simulink model "TrafficLight"  (R2021a)
settings: Solver=FixedStepDiscrete  StartTime=0.0  StopTime=inf  RelTol=1e-3
settings Model: Creator=U3  LastModifiedBy=U3
settings OptimizationCC: DefaultParameterBehavior=Inlined  EnhancedBackFolding=on  PassReuseOutputArgsAs=Individual arguments  ZeroExternalMemoryAtStartup=off  ZeroInternalMemoryAtStartup=off  OptimizeBlockOrder=speed  DifferentSizesBufferReuse=on  OptimizationCustomize=off  EfficientTunableParamExpr=on
settings DebuggingCC: UnderspecifiedInitializationDetection=Classic  MergeDetectMultiDrivingBlocksExec=none  ParameterTunabilityLossMsg=error
settings ModelReferenceCC: PropagateSignalLabelsOutOfModel=off
settings SFSimCC: MATLABDynamicMemAlloc=off
settings RTWCC: SystemTargetFile=ert.tlc  GenCodeOnly=on  TemplateMakefile=ert_default_tmf  GenerateReport=on  IncludeHyperlinkInReport=on  LaunchReport=on  GenerateTraceInfo=on  GenerateTraceReport=on  GenerateTraceReportSl=on  GenerateTraceReportSf=on  GenerateTraceReportEml=on
settings CodeAppCC: ForceParamTrailComments=on  IgnoreCustomStorageClasses=off  OperatorAnnotations=on  SimulinkDataObjDesc=on  SFDataObjDesc=on  InsertBlockDesc=on
settings ERTTargetCC: TargetLangStandard=C99 (ISO)  GenerateSampleERTMain=on  InlinedParameterPlacement=NonHierarchical  ERTCustomFileTemplate=example_file_process.tlc

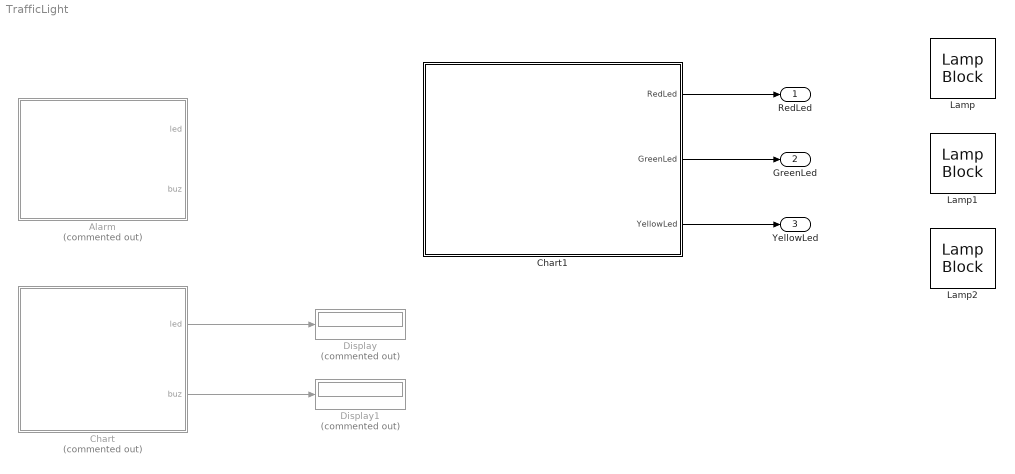
== system TrafficLight ==
  Alarm : Stateflow chart  Commented=on  TreatAsAtomicUnit=on
  Chart : Stateflow chart  Commented=on  TreatAsAtomicUnit=on
  Chart1 : Stateflow chart  TreatAsAtomicUnit=on
  Display : Display  Commented=on
  Display1 : Display  Commented=on
  Lamp : LampBlock  LabelPosition=Bottom
  Lamp1 : LampBlock  LabelPosition=Bottom
  Lamp2 : LampBlock  LabelPosition=Bottom
  RedLed : Outport
  GreenLed : Outport  Port=2
  YellowLed : Outport  Port=3
  wires:
  Chart/1(led) -> Display/1
  Chart/2(buz) -> Display1/1
  Chart1/1(RedLed) -> RedLed/1
  Chart1/2(GreenLed) -> GreenLed/1
  Chart1/3(YellowLed) -> YellowLed/1

== stateflow chart TrafficLight/Chart1 ==
  state Init
    en:
    RedLed = 0;
    GreenLed = 0;
    YellowLed = 0;
  state Red
    en:
    RedLed = 1;
    du:
    ex:
    RedLed = 0;
  state Yellow
    en:
    YellowLed = 1;
    du:
    ex:
    YellowLed = 0;
  state Green
    en:
    GreenLed = 1;
    du:
    ex:
    GreenLed = 0;
  (default) -> Init
  Init -> Red
  Yellow -> Red : [after(30, sec)]
  Red -> Green : [after(30, sec)]
  Green -> Yellow : [after(30, sec)]
  data: RedLed output [0..1] =0; GreenLed output [0..1] =0; YellowLed output [0..1] =0

== stateflow chart TrafficLight/Alarm ==
  state AlarmOFF
    en:
    flag = 0;
    count = 0;
    du:
    led = 0;
    buz = 0;
    count++;
    ex:
  state AlarmOn
    en:
    flag =  1;
    count = 0;
    du:
    led =1;
    buz = 1;
    count++;
    ex:
  (default) -> AlarmOFF
  AlarmOFF -> AlarmOn : [count == 6]
  AlarmOn -> AlarmOFF : [count == 7]
  data: flag local uint8 [0..1] =0; count local uint8 =0; led output uint8 [0..1] =0; buz output uint8 [0..1] =0

== stateflow chart TrafficLight/Chart ==
  (default) -> (junction 45) : /* Checking */
  (junction 46) -> (junction 11)
  (junction 45) -> (junction 47)
  (junction 11) -> (junction 12) [order 1] : [count < 8]
  (junction 11) -> (junction 13) [order 2]
  (junction 12) -> (junction 17) : {led = 0; buz = 0;}
  (junction 47) -> (junction 46) [order 1] : [count < 6]
  (junction 47) -> (junction 15) [order 2]
  (junction 13) -> (junction 14) [order 1] : [count == 7]
  (junction 13) -> (junction 15) [order 2] : {count++}
  (junction 14) -> (junction 16) : {led =1; buz = 1;count = 1;}
  (junction 16) -> (junction 15)
  (junction 17) -> (junction 16)
  data: flag local uint8 [0..1] =0; count local uint8 =0; led output uint8 [0..1] =0; buz output uint8 [0..1] =0
